simulink model "V4"  (R2024b)
settings: Solver=ode1  StartTime=0.0  StopTime=inf  FixedStep=0.01  RelTol=1e-3  EnableMultiTasking=on
PostLoadFcn:
  | qlabs_setup
model workspace (MAT data in the model file):
  Sig = Simulink.Signal
  Sig.Dimensions = -1
  Sig.DimensionsMode = 'auto'
  Sig.Complexity = 'auto'
  Sig.SampleTime = -1
  Sig.SamplingMode = 'auto'
  Sig.DataType = 'auto'
  downCamStepSize = Simulink.Parameter
  downCamStepSize.Value = Simulink.data.Expression
  downCamStepSize.Value.ExpressionString = "qc_get_step_size*ceil(1/30/qc_get_step_size)"
  downCamStepSize.Complexity = 'real'
  downCamStepSize.Dimensions = -1
  downCamStepSize.DataType = 'auto'
  lidarStepSize = Simulink.Parameter
  lidarStepSize.Value = Simulink.data.Expression
  lidarStepSize.Value.ExpressionString = "qc_get_step_size*ceil(1/5/qc_get_step_size)"
  lidarStepSize.Complexity = 'real'
  lidarStepSize.Dimensions = -1
  lidarStepSize.DataType = 'auto'
  mainStepSize = Simulink.Parameter
  mainStepSize.Value = Simulink.data.Expression
  mainStepSize.Value.ExpressionString = "qc_get_step_size"
  mainStepSize.Complexity = 'real'
  mainStepSize.Dimensions = -1
  mainStepSize.DataType = 'auto'
  mode = Simulink.Parameter
  mode.Value = 2
  mode.Complexity = 'real'
  mode.Dimensions = [1 1]
  mode.Description = '0 - education speeds via wheel speed commands
    | 1 - education speeds via body speed commands
    | 2 - research speeds via wheel speed commands
    | 3 - research speeds via body speed commands'
  mode.DataType = 'auto'
  realSenseStepSize = Simulink.Parameter
  realSenseStepSize.Value = Simulink.data.Expression
  realSenseStepSize.Value.ExpressionString = "qc_get_step_size*ceil(1/30/qc_get_step_size)"
  realSenseStepSize.Complexity = 'real'
  realSenseStepSize.Dimensions = -1
  realSenseStepSize.DataType = 'auto'
values from neighbouring files (symbols this model uses):
  dt = 0.01    [init.m]    (also in init1.m; init_V2.m; init_V3.m)
  map = zeros(mapHeight*pointPerMeter, mapWidth*pointPerMeter)    [map_creator.m]    (also in map_creator_real.m)
  obstacles = [obstacles; coordinateX, coordinateY, rayon;]    [init.m]    (also in init1.m; init_V2.m; init_V3.m; map_creator.m = [)
  pointPerMeter = 50    [map_creator.m]    (also in map_creator_real.m)
  Ts_mpc = 0.1    [init1.m]    (also in init_V2.m; init_V3.m)
  waypoints = [ ... (first row only)    [init.m]    (also in init1.m; init_V2.m; init_V3.m)
  x = input("Veuillez entrer la position x: ")    [map_creator_real.m]
undefined symbols (not defined in the file or in its folder): DiscIntNeverNeededParam, gcbh, JPEG, Point, qc_get_step_size, Video3D, video_display_show
libraries: quarc_library x30, mpclib x1, simulink_extras x1
(part 1 of 2)
settings Model: ExtModeTrigDuration=10000  Creator=mbohra  LastModifiedBy=toubm
settings SolverCC: PositivePriorityOrder=on  AutoInsertRateTranBlk=on
settings DebuggingCC: UnderspecifiedInitializationDetection=Classic  MergeDetectMultiDrivingBlocksExec=none
settings ModelReferenceCC: PropagateSignalLabelsOutOfModel=off
settings RTWCC: Description=QUARC Win64 Target Using Toolchain  SystemTargetFile=quarc_win64.tlc  Toolchain=QUARC win64 | nmake (64-bit Windows)  BuildConfiguration=Faster Runs  GPUComputeCapability=3.5
settings STFCustomTargetCC: TargetLangStandard=C99 (ISO)  ConcurrentExecutionCompliant=on  GRTInterface=on  UseToolchainInfoCompliant=on  SystemTargetFile=quarc_win64.tlc
settings GRTTargetCC: ParMdlRefBuildCompliant=off  CompOptLevelCompliant=off  CombineOutputUpdateFcns=off  MatFileLogging=off  CPPClassGenCompliant=off  GRTInterface=on  ExtMode=on  ExtModeMexFile=quarc_comm

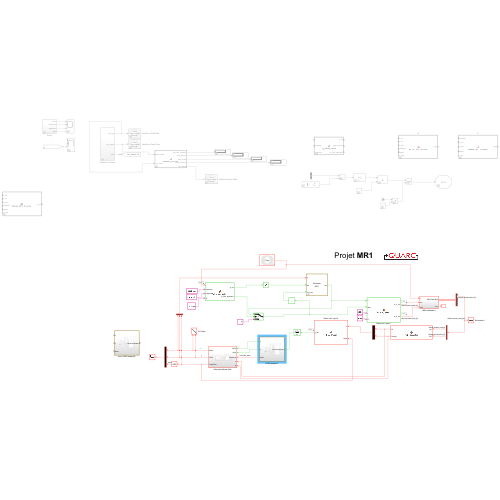
[thumbnail: Simulink's stored preview of the top-level diagram]
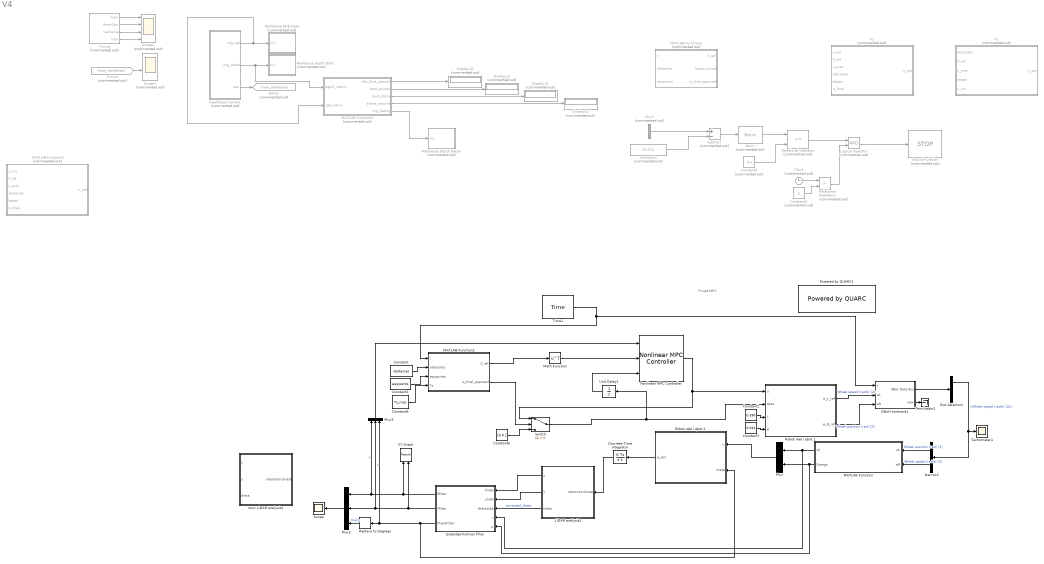
== system V4 ==
  note: Projet MR1
  Bus Selector1 : BusSelector  OutputSignals=Wheel position (rad) [2],Wheel speed (rad/s) [2],Motor Cmd (Volts) [2],Acceleration (m/s/s) [3],Gyroscope (rad/s) [3],Current (Amps) [2],Battery (Volts)
  Clock : Clock  Commented=on
  Constant : Constant  Value=obstacles  VectorParams1D=off
  Constant1 : Constant  Value=0.390
  Constant2 : Constant  Value=waypoints  VectorParams1D=off
  Constant3 : Constant  Commented=on  Value=[0,3.5]
  Constant4 : Constant  Commented=on  Value=0.3
  Constant5 : Constant  Commented=on  Value=5
  Constant6 : Constant  Value=[0 0 ]
  Constant7 : Constant  Value=0.044
  Constant8 : Constant  Value=Ts_mpc
  Demux2 : Demux  Outputs=2
  Discrete-Time Integrator : DiscreteIntegrator  SampleTime=0.1  ICPrevOutput=DiscIntNeverNeededParam  ICPrevScaledInput=DiscIntNeverNeededParam
  Display{10..13} (4 alike) : Display  Commented=on
  Extended Kalman filter : Subsystem
  From3 : From  Commented=on  GotoTag=new_realSense
  Goto2 : Goto  Commented=on  GotoTag=new_realSense
  LiDAR analysis1 : Subsystem
  Logical Operator : Logic  Commented=on  AllPortsSameDT=off  OutDataTypeStr=boolean
  MATLAB Function : MATLAB Function  TreatAsAtomicUnit=on
  MATLAB Function1 : MATLAB Function  TreatAsAtomicUnit=on  SystemSampleTime=0.1
  MATLAB Function2 : MATLAB Function  Commented=on  TreatAsAtomicUnit=on
  MATLAB Function3 : MATLAB Function  Commented=on  TreatAsAtomicUnit=on
  MATLAB Function4 : MATLAB Function  Commented=on  TreatAsAtomicUnit=on  SystemSampleTime=0.1
  Math Function : Math  Operator=transpose
  Mux : Mux  Inputs=2
  Mux1 : Mux  Commented=on  Inputs=2
  Mux2 : Mux  Inputs=3
  Mux3 : Mux  Inputs=3
  Nonlinear MPC Controller : mpclib/Nonlinear MPC Controller  nlmpcobj=nlobj  UseObjectTs=on  UseMEX=off  md_enabled=off  mvtarget_enabled=off  param_enabled=off  cost_enabled=off  mvseq_enabled=off  stateseq_enabled=off  ovseq_enabled=off  slack_enabled=off  status_enabled=off  ov_min=off  ov_max=off  mv_min=off  mv_max=off  mvrate_min=off  mvrate_max=off  state_min=off  state_max=off  ov_weight=off  mv_weight=off  mvrate_weight=off  ecr_weight=off  nlp_initialize=off
  Norm : quarc_library/Math Operations/Vectors/Norm  Commented=on
      settings: SourceProductName=QUARC Targets
  Powered by QUARC1 : quarc_library/Logos/Powered by QUARC
  QBot Hardware1 : Subsystem
  Radians to Degrees : simulink_extras/Transformations/Radians to Degrees
  RealSense Camera : Subsystem  Commented=on
  RealSense Depth Data : Subsystem  Commented=on  LoadFcn=set_param(gcbh, 'UserData', gcb);  StartFcn=video_display_show([gcb, '/Video Display'], 'add', gcb);  mask(Video Compressed Display){algorithm=JPEG, quality=50, sample_time=-1, use_hardware=on}
      mask prompts: algorithm "Compression algorithm:"; quality "Compression quality (0-100):"; sample_time "Sample time (seconds):"; use_hardware "Use hardware acceleration for video display"
      mask help: Displays a video stream on the host, using compression to minimize bandwidth.
      mask init:
      | qc_set_display('Video\nCompressed\nDisplay');
      settings: UndoDeleteFcn=set_param(gcbh, 'UserData', gcb);  OpenFcn=video_display_show([gcb, '/Video Display'], 'show', gcb);  PreDeleteFcn=video_display_show([gcb, '/Video Display'], 'delete');
      settings: CopyFcn=|
      | set_param(gcbh, 'UserData', gcb);
      | set_param(gcbh, 'LinkStatus', 'none');
      settings: NameChangeFcn=|
      | video_display_show([get_param(gcbh, 'UserData'), '/Video Display'], 'rename', [gcb, '/Video Display']);
      | video_display_show([gcb, '/Video Display'], 'add', gcb);
      | set_param(gcbh, 'UserData', gcb);
      mask Help: web(qc_get_block_help_path(gcb));
      mask TypeOptions algorithm: Image Compress/algorithm
      mask TypeOptions quality: Image Compress/quality
      mask TypeOptions sample_time: Video Display/sample_time
      mask TypeOptions use_hardware: Video Display/use_hardware
      mask Display:
      | patch([0.98591 0.98591 0.62618 0.59072 0.56147   0.536   0.536  0.5441 0.56912 0.59207 0.60881 0.62276 0.63527 0.64364  0.6485  0.6485 0.64706 0.64499 0.63662 0.62411 0.61232 0.59837 0.58307 0.56147   0.536   0.536  0.5441  0.5747 0.60953 0.63662 0.67001  0.7034 0.72851 0.75425 0.77927 0.80294 0.82454 0.84119 0.85865 0.87395 0.88574 0.89339  0.8969 0.89969 0.89969 0.89267  0.8816 0.87044 0.85649  0.8384 0.81824 0.80294 0.78764 0.77513 0.76676 0.75776 0.76397 0.77513 0.79178 0.80987 0.82796 0.84326 0.86207 0.98528],[0.18689 0.05522 0.05522 0.05171 0.05171    0.05 0.18338 0.18338 0.19148 0.20435 0.22298 0.24863 0.28589 0.33125 0.38138 0.55139 0.59801 0.63761 0.68189 0.72149 0.74939 0.76694 0.77855 0.79367 0.79952 0.92768 0.92768 0.92768 0.92417 0.92066 0.91364  0.9032 0.89384 0.88106 0.86594 0.85073 0.82634 0.80537 0.77855 0.74363 0.70403 0.65858 0.61079 0.59099 0.41513 0.37202 0.31847 0.29048 0.25556 0.23342  0.2102 0.19382 0.18221 0.17285 0.16943 0.16124  0.1589 0.16241 0.16709 0.17168  0.1787 0.18221 0.18689 0.18689],[0.9,0.90,0.91])
      | patch([0.536 0.52601 0.46823 0.44528 0.41603 0.39101 0.35555 0.33116 0.31451 0.29291  0.2804 0.26717 0.25322 0.23999 0.22406 0.20732 0.19337 0.17528 0.15935 0.14396 0.13217 0.11759 0.10922 0.10085 0.09671 0.09392 0.09041 0.08906 0.08906 0.09464  0.0995 0.10778 0.11894 0.13145 0.14675 0.16349 0.17672 0.19409 0.20732 0.22406 0.23999 0.26159 0.27833 0.29849 0.31793 0.33602 0.35411 0.37085 0.39245 0.41603   0.536   0.536 0.53159 0.46409   0.446 0.42026 0.39587 0.37571 0.36113 0.34925 0.34088 0.33809 0.33809 0.34088 0.34583 0.35627 0.36392 0.38129 0.39587 0.41117 0.42719 0.44672  0.4676 0.48353 0.48353 0.52394   0.536],[0.05 0.04829 0.04712 0.04712 0.04829 0.05063 0.05405 0.05873 0.06107 0.06692 0.07043 0.07619 0.08087 0.08672 0.09482 0.10652 0.11696 0.13325  0.1508 0.17168 0.19499 0.22415 0.25439 0.28472 0.31379 0.35456 0.38489 0.41513 0.58055 0.63878 0.68774 0.72149 0.75641 0.78089 0.80537 0.82859 0.84029 0.85658 0.86594 0.87404  0.8834 0.89267 0.90086 0.90788 0.91247 0.91832 0.92066   0.923 0.92651 0.92768 0.92768 0.79952 0.79952 0.79952 0.79718 0.78899 0.77153 0.75056 0.72149 0.68072 0.62249  0.5549 0.41396 0.37085 0.33242 0.28121 0.25205 0.22181 0.20552 0.19499 0.18572 0.18221 0.17753 0.17636 0.17753  0.1787  0.1787],[0.9,0.90,0.91])
      | disp('Video\nCompressed\nDisplay');
  RealSense Depth Data4 : Subsystem  Commented=on  LoadFcn=set_param(gcbh, 'UserData', gcb);  StartFcn=video_display_show([gcb, '/Video Display'], 'add', gcb);  mask(Video Compressed Display){algorithm=JPEG, quality=50, sample_time=-1, use_hardware=on}
      mask prompts: algorithm "Compression algorithm:"; quality "Compression quality (0-100):"; sample_time "Sample time (seconds):"; use_hardware "Use hardware acceleration for video display"
      mask help: Displays a video stream on the host, using compression to minimize bandwidth.
      mask init:
      | qc_set_display('Video\nCompressed\nDisplay');
      settings: UndoDeleteFcn=set_param(gcbh, 'UserData', gcb);  OpenFcn=video_display_show([gcb, '/Video Display'], 'show', gcb);  PreDeleteFcn=video_display_show([gcb, '/Video Display'], 'delete');
      settings: CopyFcn=|
      | set_param(gcbh, 'UserData', gcb);
      | set_param(gcbh, 'LinkStatus', 'none');
      settings: NameChangeFcn=|
      | video_display_show([get_param(gcbh, 'UserData'), '/Video Display'], 'rename', [gcb, '/Video Display']);
      | video_display_show([gcb, '/Video Display'], 'add', gcb);
      | set_param(gcbh, 'UserData', gcb);
      mask Help: web(qc_get_block_help_path(gcb));
      mask TypeOptions algorithm: Image Compress/algorithm
      mask TypeOptions quality: Image Compress/quality
      mask TypeOptions sample_time: Video Display/sample_time
      mask TypeOptions use_hardware: Video Display/use_hardware
      mask Display:
      | patch([0.98591 0.98591 0.62618 0.59072 0.56147   0.536   0.536  0.5441 0.56912 0.59207 0.60881 0.62276 0.63527 0.64364  0.6485  0.6485 0.64706 0.64499 0.63662 0.62411 0.61232 0.59837 0.58307 0.56147   0.536   0.536  0.5441  0.5747 0.60953 0.63662 0.67001  0.7034 0.72851 0.75425 0.77927 0.80294 0.82454 0.84119 0.85865 0.87395 0.88574 0.89339  0.8969 0.89969 0.89969 0.89267  0.8816 0.87044 0.85649  0.8384 0.81824 0.80294 0.78764 0.77513 0.76676 0.75776 0.76397 0.77513 0.79178 0.80987 0.82796 0.84326 0.86207 0.98528],[0.18689 0.05522 0.05522 0.05171 0.05171    0.05 0.18338 0.18338 0.19148 0.20435 0.22298 0.24863 0.28589 0.33125 0.38138 0.55139 0.59801 0.63761 0.68189 0.72149 0.74939 0.76694 0.77855 0.79367 0.79952 0.92768 0.92768 0.92768 0.92417 0.92066 0.91364  0.9032 0.89384 0.88106 0.86594 0.85073 0.82634 0.80537 0.77855 0.74363 0.70403 0.65858 0.61079 0.59099 0.41513 0.37202 0.31847 0.29048 0.25556 0.23342  0.2102 0.19382 0.18221 0.17285 0.16943 0.16124  0.1589 0.16241 0.16709 0.17168  0.1787 0.18221 0.18689 0.18689],[0.9,0.90,0.91])
      | patch([0.536 0.52601 0.46823 0.44528 0.41603 0.39101 0.35555 0.33116 0.31451 0.29291  0.2804 0.26717 0.25322 0.23999 0.22406 0.20732 0.19337 0.17528 0.15935 0.14396 0.13217 0.11759 0.10922 0.10085 0.09671 0.09392 0.09041 0.08906 0.08906 0.09464  0.0995 0.10778 0.11894 0.13145 0.14675 0.16349 0.17672 0.19409 0.20732 0.22406 0.23999 0.26159 0.27833 0.29849 0.31793 0.33602 0.35411 0.37085 0.39245 0.41603   0.536   0.536 0.53159 0.46409   0.446 0.42026 0.39587 0.37571 0.36113 0.34925 0.34088 0.33809 0.33809 0.34088 0.34583 0.35627 0.36392 0.38129 0.39587 0.41117 0.42719 0.44672  0.4676 0.48353 0.48353 0.52394   0.536],[0.05 0.04829 0.04712 0.04712 0.04829 0.05063 0.05405 0.05873 0.06107 0.06692 0.07043 0.07619 0.08087 0.08672 0.09482 0.10652 0.11696 0.13325  0.1508 0.17168 0.19499 0.22415 0.25439 0.28472 0.31379 0.35456 0.38489 0.41513 0.58055 0.63878 0.68774 0.72149 0.75641 0.78089 0.80537 0.82859 0.84029 0.85658 0.86594 0.87404  0.8834 0.89267 0.90086 0.90788 0.91247 0.91832 0.92066   0.923 0.92651 0.92768 0.92768 0.79952 0.79952 0.79952 0.79718 0.78899 0.77153 0.75056 0.72149 0.68072 0.62249  0.5549 0.41396 0.37085 0.33242 0.28121 0.25205 0.22181 0.20552 0.19499 0.18572 0.18221 0.17753 0.17636 0.17753  0.1787  0.1787],[0.9,0.90,0.91])
      | disp('Video\nCompressed\nDisplay');
  RealSense RGB Data : Subsystem  Commented=on  LoadFcn=set_param(gcbh, 'UserData', gcb);  StartFcn=video_display_show([gcb, '/Video Display'], 'add', gcb);  mask(Video Compressed Display){algorithm=JPEG, quality=50, sample_time=-1, use_hardware=on}
      mask prompts: algorithm "Compression algorithm:"; quality "Compression quality (0-100):"; sample_time "Sample time (seconds):"; use_hardware "Use hardware acceleration for video display"
      mask help: Displays a video stream on the host, using compression to minimize bandwidth.
      mask init:
      | qc_set_display('Video\nCompressed\nDisplay');
      settings: UndoDeleteFcn=set_param(gcbh, 'UserData', gcb);  OpenFcn=video_display_show([gcb, '/Video Display'], 'show', gcb);  PreDeleteFcn=video_display_show([gcb, '/Video Display'], 'delete');
      settings: CopyFcn=|
      | set_param(gcbh, 'UserData', gcb);
      | set_param(gcbh, 'LinkStatus', 'none');
      settings: NameChangeFcn=|
      | video_display_show([get_param(gcbh, 'UserData'), '/Video Display'], 'rename', [gcb, '/Video Display']);
      | video_display_show([gcb, '/Video Display'], 'add', gcb);
      | set_param(gcbh, 'UserData', gcb);
      mask Help: web(qc_get_block_help_path(gcb));
      mask TypeOptions algorithm: Image Compress/algorithm
      mask TypeOptions quality: Image Compress/quality
      mask TypeOptions sample_time: Video Display/sample_time
      mask TypeOptions use_hardware: Video Display/use_hardware
      mask Display:
      | patch([0.98591 0.98591 0.62618 0.59072 0.56147   0.536   0.536  0.5441 0.56912 0.59207 0.60881 0.62276 0.63527 0.64364  0.6485  0.6485 0.64706 0.64499 0.63662 0.62411 0.61232 0.59837 0.58307 0.56147   0.536   0.536  0.5441  0.5747 0.60953 0.63662 0.67001  0.7034 0.72851 0.75425 0.77927 0.80294 0.82454 0.84119 0.85865 0.87395 0.88574 0.89339  0.8969 0.89969 0.89969 0.89267  0.8816 0.87044 0.85649  0.8384 0.81824 0.80294 0.78764 0.77513 0.76676 0.75776 0.76397 0.77513 0.79178 0.80987 0.82796 0.84326 0.86207 0.98528],[0.18689 0.05522 0.05522 0.05171 0.05171    0.05 0.18338 0.18338 0.19148 0.20435 0.22298 0.24863 0.28589 0.33125 0.38138 0.55139 0.59801 0.63761 0.68189 0.72149 0.74939 0.76694 0.77855 0.79367 0.79952 0.92768 0.92768 0.92768 0.92417 0.92066 0.91364  0.9032 0.89384 0.88106 0.86594 0.85073 0.82634 0.80537 0.77855 0.74363 0.70403 0.65858 0.61079 0.59099 0.41513 0.37202 0.31847 0.29048 0.25556 0.23342  0.2102 0.19382 0.18221 0.17285 0.16943 0.16124  0.1589 0.16241 0.16709 0.17168  0.1787 0.18221 0.18689 0.18689],[0.9,0.90,0.91])
      | patch([0.536 0.52601 0.46823 0.44528 0.41603 0.39101 0.35555 0.33116 0.31451 0.29291  0.2804 0.26717 0.25322 0.23999 0.22406 0.20732 0.19337 0.17528 0.15935 0.14396 0.13217 0.11759 0.10922 0.10085 0.09671 0.09392 0.09041 0.08906 0.08906 0.09464  0.0995 0.10778 0.11894 0.13145 0.14675 0.16349 0.17672 0.19409 0.20732 0.22406 0.23999 0.26159 0.27833 0.29849 0.31793 0.33602 0.35411 0.37085 0.39245 0.41603   0.536   0.536 0.53159 0.46409   0.446 0.42026 0.39587 0.37571 0.36113 0.34925 0.34088 0.33809 0.33809 0.34088 0.34583 0.35627 0.36392 0.38129 0.39587 0.41117 0.42719 0.44672  0.4676 0.48353 0.48353 0.52394   0.536],[0.05 0.04829 0.04712 0.04712 0.04829 0.05063 0.05405 0.05873 0.06107 0.06692 0.07043 0.07619 0.08087 0.08672 0.09482 0.10652 0.11696 0.13325  0.1508 0.17168 0.19499 0.22415 0.25439 0.28472 0.31379 0.35456 0.38489 0.41513 0.58055 0.63878 0.68774 0.72149 0.75641 0.78089 0.80537 0.82859 0.84029 0.85658 0.86594 0.87404  0.8834 0.89267 0.90086 0.90788 0.91247 0.91832 0.92066   0.923 0.92651 0.92768 0.92768 0.79952 0.79952 0.79952 0.79718 0.78899 0.77153 0.75056 0.72149 0.68072 0.62249  0.5549 0.41396 0.37085 0.33242 0.28121 0.25205 0.22181 0.20552 0.19499 0.18572 0.18221 0.17753 0.17636 0.17753  0.1787  0.1787],[0.9,0.90,0.91])
      | disp('Video\nCompressed\nDisplay');
  Relational Operator : RelationalOperator  Commented=on  Operator=<=  OutDataTypeStr=boolean  RndMeth=Simplest  InputSameDT=off
  Relational Operator1 : RelationalOperator  Commented=on  Operator=>  OutDataTypeStr=boolean  RndMeth=Simplest  InputSameDT=off
  Robot réel / qbot 1 : MATLAB Function  TreatAsAtomicUnit=on
  Robot réel / qbot 2 : MATLAB Function  TreatAsAtomicUnit=on
  Scope : Scope
  Scope1 : Scope  Commented=on  NumInputPorts=4
  Scope2 : Scope  Commented=on  NumInputPorts=4
  Stop Simulation : Stop  Commented=on
  Subtract : Sum  Commented=on  Inputs=+-
  Switch : Switch  Criteria=u2 > Threshold  SaturateOnIntegerOverflow=off  InputSameDT=off
  Tachometer1 : Scope
  Terminator1 : Terminator
  Time1 : quarc_library/Sources/Time/Time  time_source=Wall clock  sample_time=qc_get_step_size
  Timing : Subsystem  Commented=on
  Unit Delay1 : UnitDelay  SampleTime=0.1  HasFrameUpgradeWarning=on
  V1 : MATLAB Function  Commented=on  TreatAsAtomicUnit=on
  V2 : MATLAB Function  Commented=on  TreatAsAtomicUnit=on
  XY Graph : Record  FileSettingsInternal="{\"entries\":[{\"content\":{\"excelSettings\":{\"content\":{},\"type\":\"Streamout.ExcelSettings\"}},\"type\":\"Streamout.FileSettingStorage\",\"uuid\":\"\"}],\"packageUris\":[\"http:\\/\\/schema.mathworks.com\\/mf0\\/streamout_blocks\\/R2020a\"],\"version\":\"1.0\"}"  Layout=[1 1]  SignalsInternal="{\"entries\":[{\"content\":{\"signals\":[{\"content\":{\"blockPath\":[],\"dimensions\":[1],\"domain\":\"\",\"lineColor\":\"#a2142f\",\"plots\":[ 1 ],\"port\":1,\"sid\":[\"\"],\"signalID\":1,\"signalName\":\"x\"},\"type\":\"RecordBlkView.Signal\",\"uuid\":\"\"},{\"content\":{\"blockPath\":[],\"dimensions\":[1],\"domain\":\"\",\"lineColor\":\"#139fff\",\"plots\":[ 1 ],\"port\":2,\"sid\":[\"\"],\"signalID\":2,\"signalName\":\"y\"},\"type\":\"RecordBlkView.Signal\",\"uuid\":\"\"}]},\"type\":\"RecordBlkView.InputSignals\",\"uuid\":\"\"}],\"packageUris\":[\"http:\\/\\/schema.mathworks.com\\/mf0\\/streamout_blocks\\/R2020a\"],\"version\":\"1.0\"}"  VisualizationBindings="{\"xyplotplugin\":{\"info\":[{\"series\":[{\"bindingParametersList\":[{\"parameter\":\"X-Axis\",\"signalID\":1,\"signalName\":\"x\"},{\"parameter\":\"Y-Axis\",\"signalID\":2,\"signalName\":\"y\"}],\"seriesID\":0}],\"subplotID\":1}]}}"  CompatibilityTag=XY
  nouv LiDAR analysis2 : Subsystem
  wires:
  Robot réel / qbot 2/1(q_dot) -> Discrete-Time Integrator/1
  Demux2/1 -> MATLAB Function/1(wL)  "Wheel position (rad) [2]"
  Demux2/2 -> MATLAB Function/2(wR)  "Wheel speed (rad/s) [2]"
  Constant1/1 -> Robot réel / qbot 1/3(L)
  Robot réel / qbot 1/1(w_L_ref) -> QBot Hardware1/2(wL)  "Wheel speed (rad/s) [2]"
  Time1/1 -> MATLAB Function1/1(t), QBot Hardware1/1(t)
  QBot Hardware1/2(new) -> Terminator1/1
  Bus Selector1/2 -> Demux2/1, Tachometer1/1  "<Wheel speed (rad/s) [2]>"
  QBot Hardware1/1(QBot Data Bus) -> Bus Selector1/1
  Robot réel / qbot 1/2(w_R_ref) -> QBot Hardware1/3(wR)  "Wheel position (rad) [2]"
  Constant7/1 -> Robot réel / qbot 1/4(R)
  Mux/1 -> Robot réel / qbot 2/1(u)
  Constant/1 -> MATLAB Function1/2(obstacles)
  Constant2/1 -> MATLAB Function1/3(waypoints)
  MATLAB Function1/1(X_ref) -> Math Function/1
  Mux1/1 -> Subtract/1
  Constant3/1 -> Subtract/2
  Subtract/1 -> Norm/1
  Norm/1 -> Relational Operator/1
  Constant4/1 -> Relational Operator/2
  Clock/1 -> Relational Operator1/1
  Constant5/1 -> Relational Operator1/2
  Relational Operator1/1 -> Logical Operator/2
  Relational Operator/1 -> Logical Operator/1
  Logical Operator/1 -> Stop Simulation/1
  Discrete-Time Integrator/1 -> LiDAR analysis1/1(robotCoordinate)
  MATLAB Function/2(Omega) -> Extended Kalman filter/5(w), Mux/2
  Mux2/1 -> Scope/1
  MATLAB Function/1(v0) -> Extended Kalman filter/4(v), Mux/1
  LiDAR analysis1/1(x) -> Extended Kalman filter/1(Xlidar)
  LiDAR analysis1/3(theta) -> Extended Kalman filter/3(thetaLidar)  "corrected_theta"
  Extended Kalman filter/2(Yfilter) -> Mux3/2, Mux2/2, XY Graph/2  "y"
  Extended Kalman filter/3(ThetaFilter) -> Robot réel / qbot 2/2(theta), Mux3/3, Radians to Degrees/1
  LiDAR analysis1/2(y) -> Extended Kalman filter/2(ylidar)
  Radians to Degrees/1 -> Mux2/3  "theta"
  Extended Kalman filter/1(Xfilter) -> Mux3/1, Mux2/1, XY Graph/1  "x"
  Math Function/1 -> Nonlinear MPC Controller/2
  Unit Delay1/1 -> Nonlinear MPC Controller/3
  Nonlinear MPC Controller/1 -> Switch/1, Robot réel / qbot 1/1(u)
  Mux3/1 -> Nonlinear MPC Controller/1
  RealSense Camera/2(img_depth) -> MATLAB Function3/1(depth_matrix), RealSense Depth Data/1(In1)
  RealSense Camera/3(new) -> Goto2/1
  RealSense Camera/1(img_rgb) -> RealSense RGB Data/1(In1), MATLAB Function3/2(rgb_matrix)
  MATLAB Function3/3(bord_droite) -> Display12/1
  MATLAB Function3/5(img_debug) -> RealSense Depth Data4/1(In1)
  MATLAB Function3/1(dist_face_obstacle) -> Display10/1
  MATLAB Function3/4(alerte_securite) -> Display13/1
  MATLAB Function3/2(bord_gauche) -> Display11/1
  Timing/2(downCam) -> Scope2/2
  Timing/3(realSense) -> Scope2/3
  Timing/4(lidar) -> Scope2/4
  Timing/1(main) -> Scope2/1
  From3/1 -> Scope1/3
  Constant8/1 -> MATLAB Function1/4(Ts)
  Constant6/1 -> Switch/3
  MATLAB Function1/2(is_final_approach) -> Switch/2
  Switch/1 -> Unit Delay1/1, Robot réel / qbot 1/2(data)

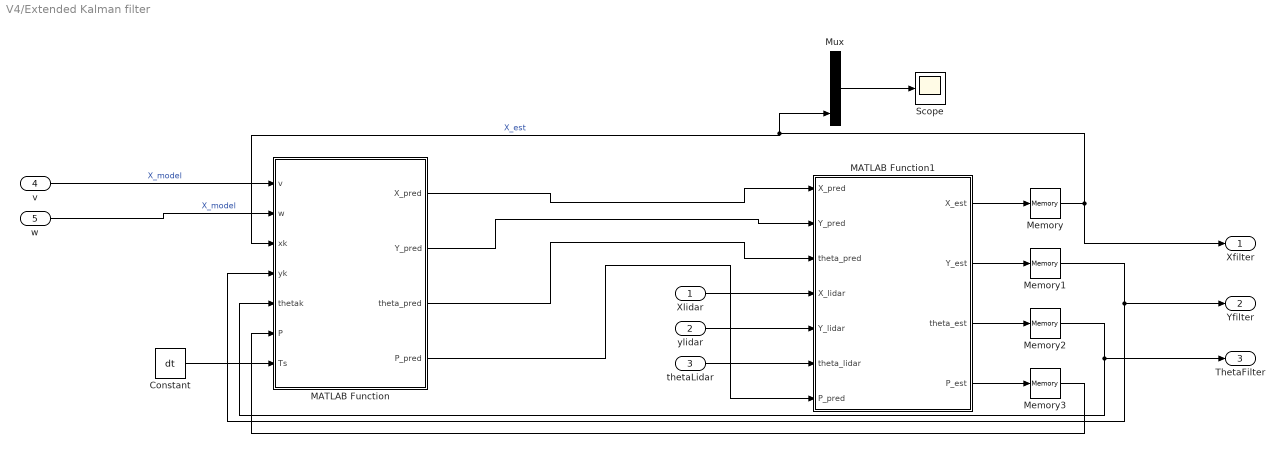
== system V4/Extended Kalman filter ==
  Xlidar : Inport
  ylidar : Inport  Port=2
  thetaLidar : Inport  Port=3
  v : Inport  Port=4
  w : Inport  Port=5
  Constant : Constant  Value=dt
  MATLAB Function : MATLAB Function  TreatAsAtomicUnit=on
  MATLAB Function1 : MATLAB Function  TreatAsAtomicUnit=on
  Memory{,1..3} (4 alike) : Memory
  Mux : Mux  Inputs=3
  Scope : Scope
  Xfilter : Outport
  Yfilter : Outport  Port=2
  ThetaFilter : Outport  Port=3
  wires:
  MATLAB Function1/3(theta_est) -> Memory2/1
  MATLAB Function/2(Y_pred) -> MATLAB Function1/2(Y_pred)
  MATLAB Function1/4(P_est) -> Memory3/1
  MATLAB Function/1(X_pred) -> MATLAB Function1/1(X_pred)
  Memory/1 -> Mux/3, MATLAB Function/3(xk), Xfilter/1  "X_est"
  Memory2/1 -> MATLAB Function/5(thetak), ThetaFilter/1
  MATLAB Function1/1(X_est) -> Memory/1
  MATLAB Function/4(P_pred) -> MATLAB Function1/7(P_pred)
  MATLAB Function/3(theta_pred) -> MATLAB Function1/3(theta_pred)
  v/1 -> MATLAB Function/1(v)  "X_model"
  Memory3/1 -> MATLAB Function/6(P)
  Memory1/1 -> MATLAB Function/4(yk), Yfilter/1
  MATLAB Function1/2(Y_est) -> Memory1/1
  Mux/1 -> Scope/1
  Xlidar/1 -> MATLAB Function1/4(X_lidar)
  ylidar/1 -> MATLAB Function1/5(Y_lidar)
  thetaLidar/1 -> MATLAB Function1/6(theta_lidar)
  w/1 -> MATLAB Function/2(w)  "X_model"
  Constant/1 -> MATLAB Function/7(Ts)

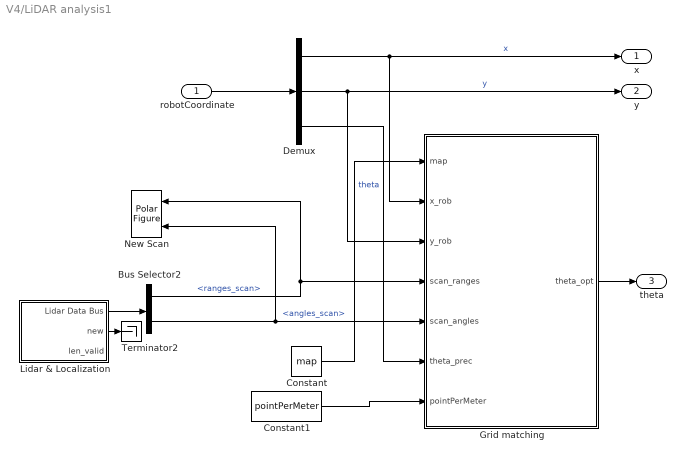
== system V4/LiDAR analysis1 ==
  robotCoordinate : Inport
  Bus Selector2 : BusSelector  OutputSignals=ranges_scan,angles_scan
  Constant : Constant  Value=map
  Constant1 : Constant  Value=pointPerMeter
  Demux : Demux  Outputs=3
  Grid matching : MATLAB Function  TreatAsAtomicUnit=on
  Lidar & Localization : Subsystem
  New Scan : quarc_library/Sinks/Figures/Polar Figure  figure_mode=Use figure window  figure_tag=figure1  axes_tag=axes1  plot_mode=Frame-based  minimum_rho=0  maximum_rho=4  minimum_theta=0  maximum_theta=360  zero_location=top  direction=counterclockwise  buffer_size=1  update_rate=1  sample_time=-1  initial_position="520  231  433  389"  initial_visibility=off  line1_style=None  line1_width=0.5  line1_color=[0 0.4470 0.7410]  marker1=Point (.)  marker1_size=6  marker1_edge_color=[0 0.447059 0.741176]  marker1_face_color=[0 0.447059 0.741176]  line2_style=Solid line (-)  line2_width=0.5  line2_color=[0.85098 0.32549 0.0980392]  marker2=None  marker2_size=6  marker2_edge_color=[0.85098 0.32549 0.0980392]  marker2_face_color=[0.85098 0.32549 0.0980392]  line3_style=Solid line (-)  line3_width=0.5  line3_color=[0.929412 0.694118 0.12549]  marker3=None  marker3_size=6  marker3_edge_color=[0.929412 0.694118 0.12549]  marker3_face_color=[0.929412 0.694118 0.12549]  line4_style=Solid line (-)  line4_width=0.5  line4_color=[0.494118 0.184314 0.556863]  marker4=None  marker4_size=6  marker4_edge_color=[0.494118 0.184314 0.556863]  marker4_face_color=[0.494118 0.184314 0.556863]  line5_style=Solid line (-)  line5_width=0.5  line5_color=[0.466667 0.67451 0.188235]  marker5=None  marker5_size=6  marker5_edge_color=[0.466667 0.67451 0.188235]  marker5_face_color=[0.466667 0.67451 0.188235]
      settings: SourceProductName=QUARC Targets
  Terminator2 : Terminator
  x : Outport
  y : Outport  Port=2
  theta : Outport  Port=3
  wires:
  Constant/1 -> Grid matching/1(map)
  Demux/2 -> Grid matching/3(y_rob), y/1  "y"
  Demux/1 -> Grid matching/2(x_rob), x/1  "x"
  robotCoordinate/1 -> Demux/1
  Grid matching/1(theta_opt) -> theta/1
  Demux/3 -> Grid matching/6(theta_prec)  "theta"
  Lidar & Localization/1(Lidar Data Bus) -> Bus Selector2/1
  Lidar & Localization/2(new) -> Terminator2/1
  Bus Selector2/2 -> Grid matching/5(scan_angles), New Scan/2  "<angles_scan>"
  Bus Selector2/1 -> Grid matching/4(scan_ranges), New Scan/1  "<ranges_scan>"
  Constant1/1 -> Grid matching/7(pointPerMeter)

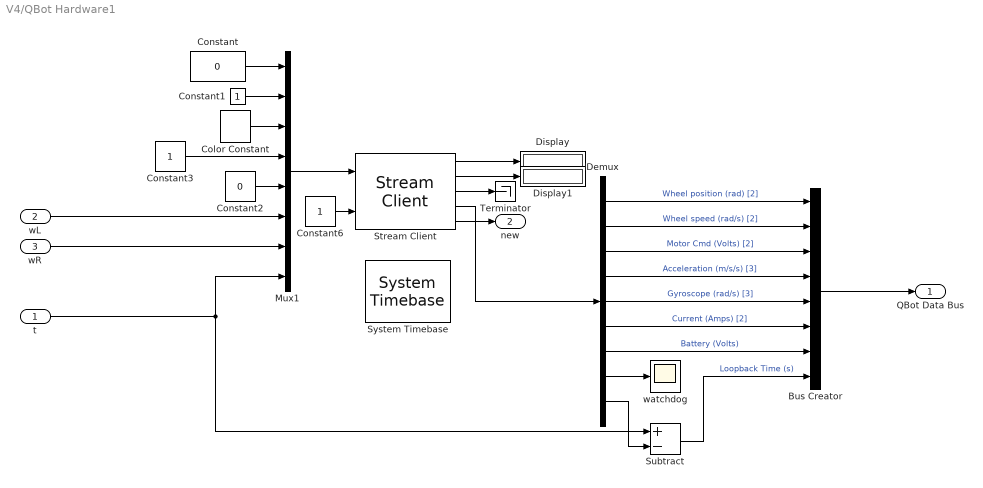
== system V4/QBot Hardware1 ==
  t : Inport
  wL : Inport  Port=2
  wR : Inport  Port=3
  Bus Creator : BusCreator  Inputs=8
  Color Constant : quarc_library/Sources/Signals/Color Constant  color=[1 0.07451 0.65098]
      settings: SourceProductName=QUARC Targets
  Constant : Constant  Value=0
  Constant1 : Constant
  Constant2 : Constant  Value=0
  Constant3 : Constant
  Constant6 : Constant
  Demux : Demux  Outputs=[2 2 2 3 3 2 1 1 1]
  Display : Display
  Display1 : Display
  Mux1 : Mux  Inputs=8
  Stream Client : quarc_library/Communications/Basic/Stream Client  uri_source=Specify via dialog (do not evaluate)  uri=tcpip://localhost:18888  send_buffer_size=1460  receive_buffer_size=1460  byte_order=little endian (Intel - LSB first)  optimization=Minimum latency  send_options=Send most recent data  receive_options=Receive most recent data  default_value=zeros(17,1)  sample_time=qc_get_step_size  active=on  implementation=Use blocking I/O in a separate thread  send_fifo_size=1000  receive_fifo_size=1000  send_priority=0  receive_priority=0  send_dimensions=off  receive_dimensions=off  max_dimensions=-1  data_type=Inherited via back propagation  type_expr=BusObject
      settings: AttributesFormatString="\"tcpip://localhost:18888\""
  Subtract : Sum  Inputs=+-
  System Timebase : quarc_library/Advanced/Timing/System Timebase  stop_on_overrun=off
      settings: SourceProductName=QUARC Targets
  Terminator : Terminator
  watchdog : Scope
  QBot Data Bus : Outport
  new : Outport  Port=2
  wires:
  Demux/2 -> Bus Creator/2  "Wheel speed (rad/s) [2]"
  Constant/1 -> Mux1/1
  Stream Client/3 -> Terminator/1
  Stream Client/1 -> Display/1
  Constant6/1 -> Stream Client/2
  Stream Client/2 -> Display1/1
  Color Constant/1 -> Mux1/3
  Constant1/1 -> Mux1/2
  Demux/3 -> Bus Creator/3  "Motor Cmd (Volts) [2]"
  Mux1/1 -> Stream Client/1
  Stream Client/4 -> Demux/1
  Demux/1 -> Bus Creator/1  "Wheel position (rad) [2]"
  Stream Client/5 -> new/1
  Demux/7 -> Bus Creator/7  "Battery (Volts)"
  Demux/5 -> Bus Creator/5  "Gyroscope (rad/s) [3]"
  Demux/6 -> Bus Creator/6  "Current (Amps) [2]"
  Demux/9 -> Subtract/2
  Constant2/1 -> Mux1/5
  Demux/4 -> Bus Creator/4  "Acceleration (m/s/s) [3]"
  t/1 -> Subtract/1, Mux1/8
  Bus Creator/1 -> QBot Data Bus/1
  Subtract/1 -> Bus Creator/8  "Loopback Time (s)"
  Demux/8 -> watchdog/1
  Constant3/1 -> Mux1/4
  wL/1 -> Mux1/6
  wR/1 -> Mux1/7

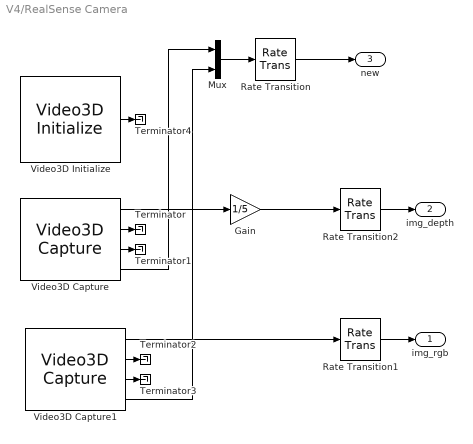
== system V4/RealSense Camera ==
  Gain : Gain  Gain=1/5
  Mux : Mux  Inputs=2
  Rate Transition : RateTransition
  Rate Transition1 : RateTransition  OutPortSampleTime=realSenseStepSize*2
  Rate Transition2 : RateTransition  OutPortSampleTime=realSenseStepSize*2
  Terminator{,1..4} (5 alike) : Terminator
  Video3D Capture : quarc_library/Multimedia/Video3D Capture  object_name=Video3D-1  stream_type=Depth  stream_index=0  resolution=640 x 480  width=640  height=480  output_format=Distance in meters (HxW)  data_type=single  sample_time=realSenseStepSize  camera_intrinsics=off  depth_scale=off  brightness_override=Do not override  brightness=50.0  contrast_override=Do not override  contrast=50.0  hue_override=Do not override  hue=50.0  saturation_override=Do not override  saturation=50.0  sharpness_override=Do not override  sharpness=50.0  gamma_override=Do not override  gamma=50.0  gain_override=Do not override  gain=50.0  backlightcompensation_override=Do not override  backlightcompensation=50.0  whitebalance_override=Automatic white balance  whitebalance=50.0  exposure_override=Automatic exposure  exposure=30.0  emitter=Enable laser emitter  preset=Do not set camera presets
  Video3D Capture1 : quarc_library/Multimedia/Video3D Capture  object_name=Video3D-1  stream_type=RGB  stream_index=0  resolution=640 x 480  width=640  height=480  output_format=MATLAB RGB (HxWx3)  data_type=uint8  sample_time=realSenseStepSize  camera_intrinsics=off  depth_scale=off  brightness_override=Do not override  brightness=50.0  contrast_override=Do not override  contrast=50.0  hue_override=Do not override  hue=50.0  saturation_override=Do not override  saturation=50.0  sharpness_override=Do not override  sharpness=50.0  gamma_override=Do not override  gamma=50.0  gain_override=Do not override  gain=50.0  backlightcompensation_override=Do not override  backlightcompensation=50.0  whitebalance_override=Automatic white balance  whitebalance=50.0  exposure_override=Automatic exposure  exposure=30.0  emitter=Enable laser emitter  preset=Do not set camera presets
  Video3D Initialize : quarc_library/Multimedia/Video3D Initialize  object_name=Video3D-1  source=Device  identifier=0@tcpip://localhost:18917  file=sample.bag  sample_time=qc_get_step_size *2  active=on
  img_rgb : Outport
  img_depth : Outport  Port=2
  new : Outport  Port=3
  wires:
  Video3D Capture1/1 -> Rate Transition1/1
  Mux/1 -> Rate Transition/1
  Video3D Capture/4 -> Mux/1
  Video3D Capture1/4 -> Mux/2
  Video3D Capture/2 -> Terminator/1
  Video3D Capture/3 -> Terminator1/1
  Video3D Capture1/2 -> Terminator2/1
  Video3D Capture1/3 -> Terminator3/1
  Video3D Initialize/1 -> Terminator4/1
  Rate Transition/1 -> new/1
  Rate Transition1/1 -> img_rgb/1
  Rate Transition2/1 -> img_depth/1
  Video3D Capture/1 -> Gain/1
  Gain/1 -> Rate Transition2/1

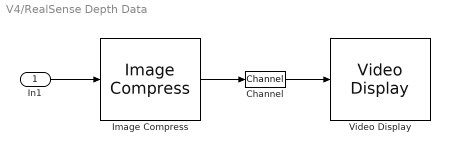
== system V4/RealSense Depth Data ==
  In1 : Inport
  Channel : quarc_library/Signal Routing/Channel  channel=0  buffer_size=1
  Image Compress : quarc_library/Image Processing/Generic/Image Compress  algorithm=JPEG  source=Internal dialog parameter  quality=quality  output_dim=-1
  Video Display : quarc_library/Multimedia/Video Display  Tag=fusion_des_travaux_bloc_NMPC_MATLAB_V2_TEST_AVEC_CAM_test/RealSense Depth Data/Video Display  sample_time=sample_time  use_hardware=on
  wires:
  Channel/1 -> Video Display/1
  In1/1 -> Image Compress/1
  Image Compress/1 -> Channel/1

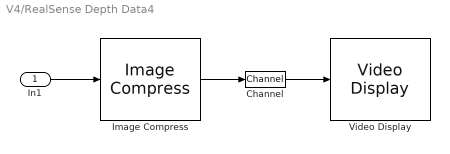
== system V4/RealSense Depth Data4 ==
  In1 : Inport
  Channel : quarc_library/Signal Routing/Channel  channel=1  buffer_size=1
  Image Compress : quarc_library/Image Processing/Generic/Image Compress  algorithm=JPEG  source=Internal dialog parameter  quality=quality  output_dim=-1
  Video Display : quarc_library/Multimedia/Video Display  Tag=fusion_des_travaux_bloc_NMPC_MATLAB_V2_TEST_AVEC_CAM_test/RealSense Depth Data4/Video Display  sample_time=sample_time  use_hardware=on
  wires:
  Channel/1 -> Video Display/1
  In1/1 -> Image Compress/1
  Image Compress/1 -> Channel/1

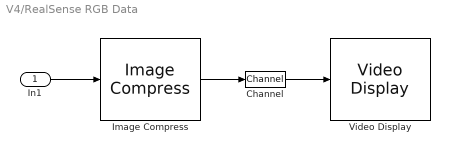
== system V4/RealSense RGB Data ==
  In1 : Inport
  Channel : quarc_library/Signal Routing/Channel  channel=2  buffer_size=1
  Image Compress : quarc_library/Image Processing/Generic/Image Compress  algorithm=JPEG  source=Internal dialog parameter  quality=quality  output_dim=-1
  Video Display : quarc_library/Multimedia/Video Display  Tag=fusion_des_travaux_bloc_NMPC_MATLAB_V2_TEST_AVEC_CAM_test/RealSense RGB Data/Video Display  sample_time=sample_time  use_hardware=on
  wires:
  Image Compress/1 -> Channel/1
  In1/1 -> Image Compress/1
  Channel/1 -> Video Display/1

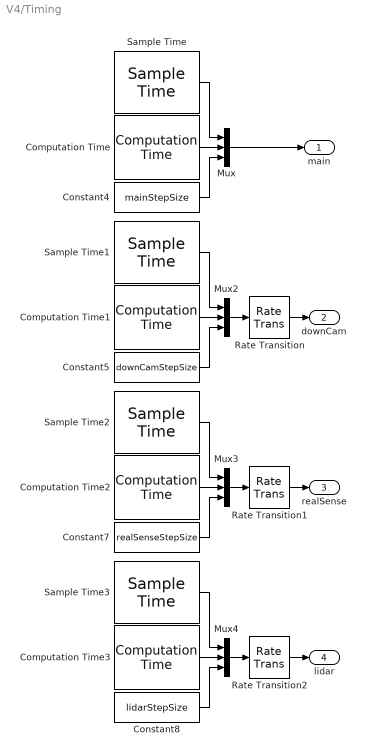
== system V4/Timing ==
  Computation Time : quarc_library/Sources/Time/Computation Time  sample_time=mainStepSize  use_model=on  use_cpu_time=off
  Computation Time1 : quarc_library/Sources/Time/Computation Time  sample_time=downCamStepSize  use_model=on  use_cpu_time=off
  Computation Time2 : quarc_library/Sources/Time/Computation Time  sample_time=realSenseStepSize  use_model=on  use_cpu_time=off
  Computation Time3 : quarc_library/Sources/Time/Computation Time  sample_time=lidarStepSize  use_model=on  use_cpu_time=off
  Constant4 : Constant  Value=mainStepSize
  Constant5 : Constant  Value=downCamStepSize
  Constant7 : Constant  Value=realSenseStepSize
  Constant8 : Constant  Value=lidarStepSize
  Mux{,2..4} (4 alike) : Mux  Inputs=3
  Rate Transition : RateTransition
  Rate Transition1 : RateTransition
  Rate Transition2 : RateTransition
  Sample Time : quarc_library/Sources/Time/Sample Time  Priority=-99  sample_time=mainStepSize
  Sample Time1 : quarc_library/Sources/Time/Sample Time  Priority=-99  sample_time=downCamStepSize
  Sample Time2 : quarc_library/Sources/Time/Sample Time  Priority=-99  sample_time=realSenseStepSize
  Sample Time3 : quarc_library/Sources/Time/Sample Time  Priority=-99  sample_time=lidarStepSize
  main : Outport
  downCam : Outport  Port=2
  realSense : Outport  Port=3
  lidar : Outport  Port=4
  wires:
  Rate Transition1/1 -> realSense/1
  Computation Time2/1 -> Mux3/2
  Constant5/1 -> Mux2/3
  Mux4/1 -> Rate Transition2/1
  Computation Time/1 -> Mux/2
  Sample Time/1 -> Mux/1
  Constant8/1 -> Mux4/3
  Sample Time1/1 -> Mux2/1
  Mux3/1 -> Rate Transition1/1
  Computation Time1/1 -> Mux2/2
  Constant4/1 -> Mux/3
  Mux2/1 -> Rate Transition/1
  Computation Time3/1 -> Mux4/2
  Sample Time2/1 -> Mux3/1
  Constant7/1 -> Mux3/3
  Sample Time3/1 -> Mux4/1
  Rate Transition/1 -> downCam/1
  Rate Transition2/1 -> lidar/1
  Mux/1 -> main/1

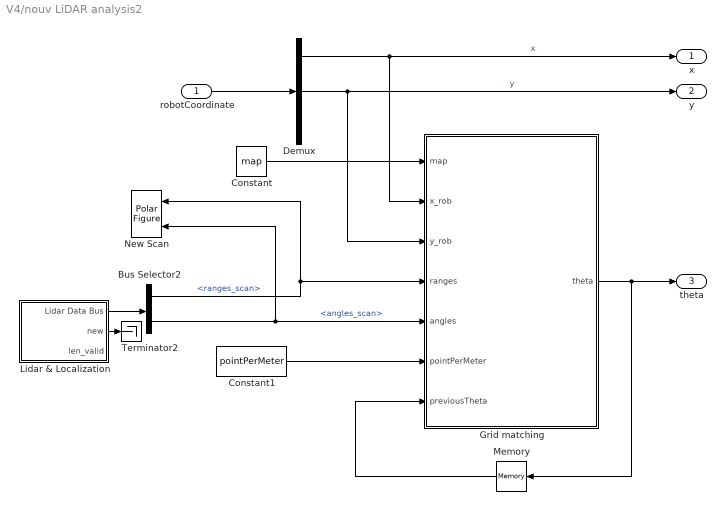
== system V4/nouv LiDAR analysis2 ==
  robotCoordinate : Inport
  Bus Selector2 : BusSelector  OutputSignals=ranges_scan,angles_scan
  Constant : Constant  Value=map
  Constant1 : Constant  Value=pointPerMeter
  Demux : Demux  Outputs=3
  Grid matching : MATLAB Function  TreatAsAtomicUnit=on
  Lidar & Localization : Subsystem
  Memory : Memory
  New Scan : quarc_library/Sinks/Figures/Polar Figure  figure_mode=Use figure window  figure_tag=figure1  axes_tag=axes1  plot_mode=Frame-based  minimum_rho=0  maximum_rho=4  minimum_theta=0  maximum_theta=360  zero_location=top  direction=counterclockwise  buffer_size=1  update_rate=1  sample_time=-1  initial_position="520  231  433  389"  initial_visibility=off  line1_style=None  line1_width=0.5  line1_color=[0 0.4470 0.7410]  marker1=Point (.)  marker1_size=6  marker1_edge_color=[0 0.447059 0.741176]  marker1_face_color=[0 0.447059 0.741176]  line2_style=Solid line (-)  line2_width=0.5  line2_color=[0.85098 0.32549 0.0980392]  marker2=None  marker2_size=6  marker2_edge_color=[0.85098 0.32549 0.0980392]  marker2_face_color=[0.85098 0.32549 0.0980392]  line3_style=Solid line (-)  line3_width=0.5  line3_color=[0.929412 0.694118 0.12549]  marker3=None  marker3_size=6  marker3_edge_color=[0.929412 0.694118 0.12549]  marker3_face_color=[0.929412 0.694118 0.12549]  line4_style=Solid line (-)  line4_width=0.5  line4_color=[0.494118 0.184314 0.556863]  marker4=None  marker4_size=6  marker4_edge_color=[0.494118 0.184314 0.556863]  marker4_face_color=[0.494118 0.184314 0.556863]  line5_style=Solid line (-)  line5_width=0.5  line5_color=[0.466667 0.67451 0.188235]  marker5=None  marker5_size=6  marker5_edge_color=[0.466667 0.67451 0.188235]  marker5_face_color=[0.466667 0.67451 0.188235]
      settings: SourceProductName=QUARC Targets
  Terminator2 : Terminator
  x : Outport
  y : Outport  Port=2
  theta : Outport  Port=3
  wires:
  Constant/1 -> Grid matching/1(map)
  Demux/2 -> Grid matching/3(y_rob), y/1  "y"
  Demux/1 -> Grid matching/2(x_rob), x/1  "x"
  robotCoordinate/1 -> Demux/1
  Grid matching/1(theta) -> theta/1, Memory/1
  Lidar & Localization/1(Lidar Data Bus) -> Bus Selector2/1
  Lidar & Localization/2(new) -> Terminator2/1
  Bus Selector2/2 -> Grid matching/5(angles), New Scan/2  "<angles_scan>"
  Bus Selector2/1 -> Grid matching/4(ranges), New Scan/1  "<ranges_scan>"
  Constant1/1 -> Grid matching/6(pointPerMeter)
  Memory/1 -> Grid matching/7(previousTheta)

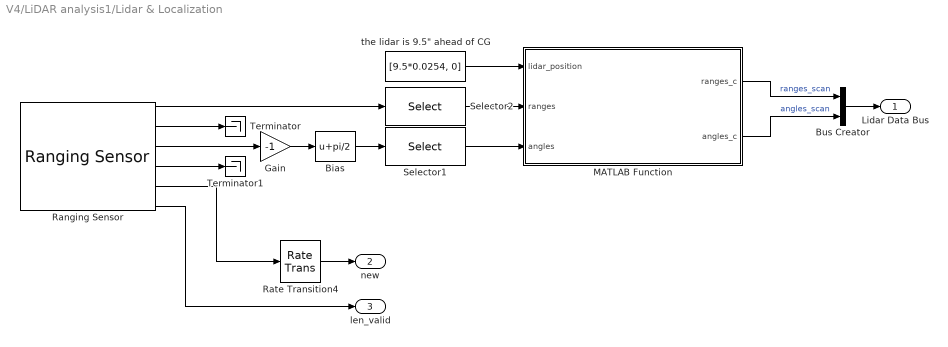
== system V4/LiDAR analysis1/Lidar & Localization ==
  Bias : Bias  Bias=pi/2  SaturateOnIntegerOverflow=off
  Bus Creator : BusCreator  Inputs=2
  Gain : Gain  Gain=-1
  MATLAB Function : MATLAB Function  TreatAsAtomicUnit=on
  Ranging Sensor : quarc_library/Devices/Third-Party/Sensors/Ranging Sensor  sensor_type=Leishen M10P LIDAR  uri=tcpip://localhost:18918  ranging_distance=Short  timing_budget=0.033  measurement_period=0.0005  output_mode=Fixed-size output  samples_per_revolution=1680  max_distance=0.050  max_angle=5  sample_time=lidarStepSize  show_versions=off  active=on
      settings: SourceProductName=QUARC Targets
  Rate Transition4 : RateTransition
  Selector1 : Selector  InputPortWidth=1680  IndexOptions=Index vector (dialog)  Indices=[1:4:1677]  OutputSizes=1
  Selector2 : Selector  InputPortWidth=1680  IndexOptions=Index vector (dialog)  Indices=[1:4:1677]  OutputSizes=1
  Terminator : Terminator
  Terminator1 : Terminator
  "the lidar is 9.5\" ahead of CG" : Constant  Value=[9.5*0.0254, 0]  SampleTime=lidarStepSize
  Lidar Data Bus : Outport
  new : Outport  Port=2
  len_valid : Outport  Port=3
  wires:
  Ranging Sensor/5 -> Rate Transition4/1
  Rate Transition4/1 -> new/1
  Selector1/1 -> MATLAB Function/3(angles)
  Selector2/1 -> MATLAB Function/2(ranges)
  "the lidar is 9.5\" ahead of CG"/1 -> MATLAB Function/1(lidar_position)
  Bias/1 -> Selector1/1
  Ranging Sensor/2 -> Terminator/1
  Ranging Sensor/4 -> Terminator1/1
  Gain/1 -> Bias/1
  Ranging Sensor/3 -> Gain/1
  Ranging Sensor/1 -> Selector2/1
  MATLAB Function/1(ranges_c) -> Bus Creator/1  "ranges_scan"
  MATLAB Function/2(angles_c) -> Bus Creator/2  "angles_scan"
  Bus Creator/1 -> Lidar Data Bus/1
  Ranging Sensor/6 -> len_valid/1

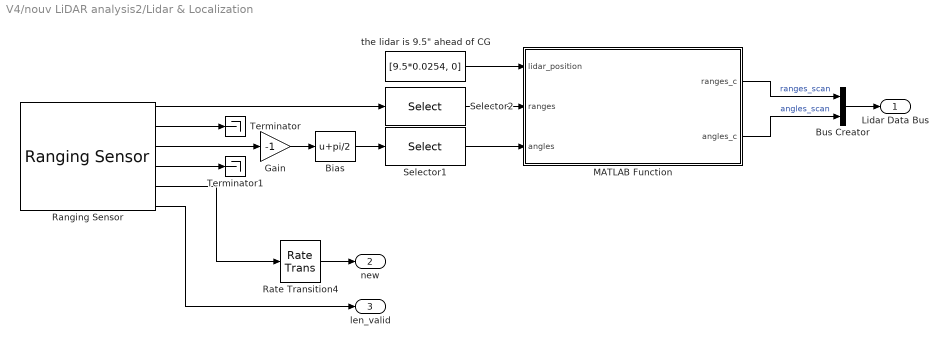
== system V4/nouv LiDAR analysis2/Lidar & Localization ==
  Bias : Bias  Bias=pi/2  SaturateOnIntegerOverflow=off
  Bus Creator : BusCreator  Inputs=2
  Gain : Gain  Gain=-1
  MATLAB Function : MATLAB Function  TreatAsAtomicUnit=on
  Ranging Sensor : quarc_library/Devices/Third-Party/Sensors/Ranging Sensor  sensor_type=Leishen M10P LIDAR  uri=tcpip://localhost:18918  ranging_distance=Short  timing_budget=0.033  measurement_period=0.0005  output_mode=Fixed-size output  samples_per_revolution=1680  max_distance=0.050  max_angle=5  sample_time=lidarStepSize  show_versions=off  active=on
      settings: SourceProductName=QUARC Targets
  Rate Transition4 : RateTransition
  Selector1 : Selector  InputPortWidth=1680  IndexOptions=Index vector (dialog)  Indices=[1:4:1677]  OutputSizes=1
  Selector2 : Selector  InputPortWidth=1680  IndexOptions=Index vector (dialog)  Indices=[1:4:1677]  OutputSizes=1
  Terminator : Terminator
  Terminator1 : Terminator
  "the lidar is 9.5\" ahead of CG" : Constant  Value=[9.5*0.0254, 0]  SampleTime=lidarStepSize
  Lidar Data Bus : Outport
  new : Outport  Port=2
  len_valid : Outport  Port=3
  wires:
  Ranging Sensor/5 -> Rate Transition4/1
  Rate Transition4/1 -> new/1
  Selector1/1 -> MATLAB Function/3(angles)
  Selector2/1 -> MATLAB Function/2(ranges)
  "the lidar is 9.5\" ahead of CG"/1 -> MATLAB Function/1(lidar_position)
  Bias/1 -> Selector1/1
  Ranging Sensor/2 -> Terminator/1
  Ranging Sensor/4 -> Terminator1/1
  Gain/1 -> Bias/1
  Ranging Sensor/3 -> Gain/1
  Ranging Sensor/1 -> Selector2/1
  MATLAB Function/1(ranges_c) -> Bus Creator/1  "ranges_scan"
  MATLAB Function/2(angles_c) -> Bus Creator/2  "angles_scan"
  Bus Creator/1 -> Lidar Data Bus/1
  Ranging Sensor/6 -> len_valid/1

== matlab function V4/Extended Kalman filter/MATLAB Function1 ==
  data: X_pred input; X_est output; Y_pred input; theta_pred input; X_lidar input; Y_lidar input; theta_lidar input; P_pred input; Y_est output; theta_est output; P_est output
function [X_est, Y_est, theta_est, P_est] = update(X_pred, Y_pred, theta_pred, X_lidar, Y_lidar, theta_lidar, P_pred)
    % 1. VECTEURS D'ÉTAT ET DE MESURE
    x_p = [X_pred; Y_pred; theta_pred];
    z = [X_lidar; Y_lidar; theta_lidar];

    % 2. MODÈLE D'OBSERVATION (H)
    % Puisque le LIDAR mesure directement x, y et theta, H est l'identité
    H = eye(3);

    % 3. MATRICE DE BRUIT DE MESURE (R)
    % Plus ces valeurs sont faibles, plus le filtre fera confiance au LIDAR
    % (À ajuster selon la précision du LIDAR)
    r_dist = 0.05; %0.00005; % Incertitude en mètres 0.05
    r_ang  = 0.05; %0.00002; % Incertitude en radians0.02
    R = diag([r_dist, r_dist, r_ang]);

    % 4. CALCUL DU GAIN DE KALMAN (K)
    % S est la covariance de l'innovation
    S = H * P_pred * H' + R;
    K = P_pred * H' / S;

    % 5. CALCUL DE L'Erreur entre LIDAR et Prédiction
    innovation = z - (H * x_p);

    %Normalisation de l'erreur d'angle
    % Empêche le filtre de paniquer si le LIDAR dit 179° et le modèle 181° (-179°)
    innovation(3) = atan2(sin(innovation(3)), cos(innovation(3)));

    % 6. MISE À JOUR DE L'ÉTAT ET DE LA COVARIANCE
    x_corrected = x_p + K * innovation;
    %P_corrected = (eye(3) - K * H) * P_pred;
    IKH = eye(3) - K * H;
    P_corrected = IKH * P_pred * IKH' + K * R * K';

    % 7. ASSIGNATION DES SORTIES
    X_est = x_corrected(1);
    Y_est = x_corrected(2);
    % theta_est = atan2(sin(x_corrected(3)), cos(x_corrected(3)));
    theta_est = atan2(sin(x_corrected(3)), cos(x_corrected(3))); % CHNGEMENTNNNTNNTNTNN
    %theta_est = x_corrected(3);
    P_est = P_corrected;
end

== matlab function V4/nouv LiDAR analysis2/Lidar & Localization/MATLAB Function ==
  data: lidar_position input; ranges input; ranges_c output; angles input; angles_c output
function [ranges_c,angles_c] = correct_lidar(lidar_position, ranges,angles)

x = ranges.*cos(angles) + lidar_position(1);
y = ranges.*sin(angles) + lidar_position(2);

ranges_c = sqrt(x.^2 + y.^2);
angles_c = atan2(y, x);

end

== matlab function V4/MATLAB Function4 ==
  data: x_init input size=[3,1]; X_ref input size=[3, 25]; u_prev input; obstacles input; u_opt output; kappa input; is_final input
function u_opt = Matisse_MPC_Quanser(x_init, X_ref, u_prev, obstacles, kappa, is_final)
    % Entrées :
    %   x_init    : État courant [x; y; theta] — position RÉELLE mesurée
    %   X_ref     : Références futures [3 x Np]
    %   u_prev    : Commande précédente [v; omega]
    %   obstacles : Obstacles circulaires [x, y, rayon]
    %   kappa     : Courbure locale courante
    %   is_final  : Flag d'approche finale (0 ou 1)

    coder.extrinsic('solve_mpc_matisse');

    % --- Paramètres ---
    Np    = 25;
    Ts    = 0.1;
    v_max = 0.5;
    w_max = 2.0;

    % Rayon d'arrêt : distance réelle robot -> goal en dessous de laquelle on stoppe
    STOP_RADIUS = 0.12;

    % Pre-allocation obligatoire sinon  Simulink galère
    u_seq = zeros(2*Np, 1);
    u_opt = zeros(2, 1);
    goal_pos   = X_ref(1:2, end);
    robot_pos  = x_init(1:2);
    dist_final = norm(robot_pos - goal_pos);

    persistent stop_locked
    if isempty(stop_locked)
        stop_locked = int32(0);
    end

    % On verrouille des qu'on est dans le rayon d'arret ET en approche finale
    if is_final == 1 && dist_final < STOP_RADIUS
        stop_locked = int32(1);
    end

    if stop_locked == 1
        u_opt = [0; 0];
        return;
    end

    % --- Matrices de Ponderation de base ---
    Q = diag([10, 10, 1.0]); % angle 10x plus penalise pour eviter rotation en rond
    R = diag([0.1, 0.1]);
    S = diag([1, 8]); %penalite omega augmentee pour eviter oscillations angulaires

    % ORDRE P=Q : on modifie Q AVANT de copier dans P
    if is_final == 1
        % En approche finale : on augmente la penalite de position
        % et on relache l'angle pour eviter le vrillage
        Q(1,1) = 30;
        Q(2,2) = 30;
        Q(3,3) = 0.01;

        % =========================================================
        % ANTI-DEPASSEMENT : si le robot est presque perpendiculaire
        % ou dos au goal, on reduit v_max pour freiner.
        % Produit scalaire vecteur robot->goal vs direction courante.
        % =========================================================
        vec_to_goal = goal_pos - robot_pos;
        heading_vec = [cos(x_init(3)); sin(x_init(3))];
        dot_product = dot(vec_to_goal / (norm(vec_to_goal) + 1e-6), heading_vec);

        if dot_product < 0.3
            % Robot presque perpendiculaire ou dos au goal -> frein fort
            v_max = 0.1;
        elseif dist_final < 0.4
            % Freinage progressif dans les 40 derniers cm
            v_max = max(0.05, v_max * (dist_final / 0.4));
        end
    end

    % P = Q apres toutes les modifications
    P = Q;

    lb = repmat([-v_max; -w_max], Np, 1);
    ub = repmat([ v_max;  w_max], Np, 1);

    % on part de u_prev repete sur tout l'horizon
    % si u_prev est nul (demarrage), on force une vitesse initiale pour que fmincon parte d'un point non-degenere
    if norm(u_prev) < 1e-6
        u0 = repmat([0.1; 0.0], Np, 1);
    else
        u0 = repmat(u_prev, Np, 1);
    end

    % Appel optimiseur
    u_seq = solve_mpc_matisse(x_init, X_ref, u_prev, Q, R, S, P, Np, Ts, obstacles, lb, ub, u0);
    u_opt = u_seq(1:2);
end

== matlab function V4/MATLAB Function ==
  data: wL input; v0 output; wR input; Omega output
function [v0, Omega] = Fwd_Kinematics(wL, wR)
    % wL : Vitesse angulaire roue gauche (rad/s)
    % wR : Vitesse angulaire roue droite (rad/s)
    % R  : Rayon de la roue (m)
    % L  : Entraxe (distance entre les roues en m)

    R = 0.044;   % Rayon de la roue (44 mm)
    L = 0.390;   % Entraxe entre les roues (39 cm)

    % 1. Conversion en vitesse linéaire de chaque roue (m/s)
    v_left = wL * R;
    v_right = wR * R;

    % 2. Calcul de la vitesse linéaire du robot (v0)
    % C'est la moyenne des deux roues
    v0 = (v_right + v_left) / 2;

    % 3. Calcul de la vitesse de rotation du robot (Omega)
    % C'est la différence de vitesse divisée par la largeur du robot
    Omega = (v_right - v_left) / L;
    
end

== matlab function V4/Robot réel // qbot 1 ==
  data: w_L_ref output; u input; data input; w_R_ref output; L input; R input
function [w_L_ref, w_R_ref] = Motors_Speed(u, data, L, R)
    % u(1) = u1 (Vitesse linéaire v en m/s)
    % u(2) = u2 (Vitesse angulaire omega en rad/s)

    v = u(1);
    omega = u(2);

    % Calcul des vitesses linéaires de chaque roue 
    w_L_ref = (2*v-L*omega)/(2*R);
    w_R_ref = (2*v+L*omega)/(2*R);
    % Conversion en vitesse angulaire (rad/s) pour les moteurs
    %w_R_ref = (v_R / R);
    %w_L_ref = (v_L / R);
end

== matlab function V4/Robot réel // qbot 2 ==
  data: u input; q_dot output; theta input
function q_dot  = Robot_Model(u, theta)
    % u(1) = u1 (vitesse linéaire)
    % u(2) = u2 (vitesse angulaire)

    q_dot = [0;0;0];
    q_dot(1) = u(1) * cos(theta);
    q_dot(2) = u(1) * sin(theta);
    q_dot(3) = u(2);
end
